simulink model "Ex4_IC"  (R2021a)
settings: Solver=VariableStepAuto  StartTime=0.0  StopTime=10.0  RelTol=1e-3
undefined symbols (not defined in the file): fdesignblkfcn, gcbh
libraries: dsparch4 x1
settings Model: Creator=gferr  LastModifiedBy=gferr

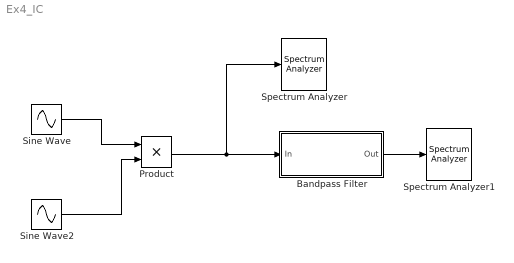
== system Ex4_IC ==
  Bandpass Filter : Subsystem  DialogController=fdesignblkfcn  InitFcn=fdesignblkfcn(gcbh, {'InitFcn'});  mask(Bandpass Filter){}
      mask help: Design a bandpass filter
      settings: CopyFcn=fdesignblkfcn(gcbh, {'CopyFcn'});
      mask Help: helpview(mapfilelocation('dsp'), 'dspbandpassfilter');
      mask Display: disp('Bandpass');
  Product : Product
  Sine Wave : Sin  Frequency=20e9  SampleTime=5e-11
  Sine Wave2 : Sin  Frequency=3.5e9  SampleTime=5e-11
  Spectrum Analyzer : SpectrumAnalyzer
  Spectrum Analyzer1 : SpectrumAnalyzer
  wires:
  Product/1 -> Bandpass Filter/1(In), Spectrum Analyzer/1
  Sine Wave2/1 -> Product/2
  Sine Wave/1 -> Product/1
  Bandpass Filter/1(Out) -> Spectrum Analyzer1/1

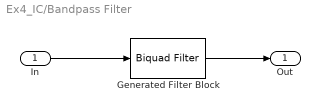
== system Ex4_IC/Bandpass Filter ==
  In : Inport
  Generated Filter Block : dsparch4/Biquad Filter  Tag=BlockMethodSubSystem  FilterSource=Dialog parameters  CoeffSource=Specify via dialog  FilterObject=BQF  IIRFiltStruct=Direct form II  BiQuadCoeffs=[0.00966146652633205656 0 -0.00966146652633205656 1 -0.893732410630936891 0.984405274774847627;0.00330714192391191354 0 -0.00330714192391191354 1 -0.880244202993088365 0.984346529334988007;0.0166040427440116885 0 -0.0166040427440116885 1 -0.907405547432020732 0.996135049550237905;0.0114751093240028565 0 -0.0114751093240028565 1 -0.876964852267980266 0.996102065629321465;0.00541103985322967471 0 -0.00541103985322967471 1 -0.886239861407497886 0.982673189944245795;0.0145645545686283809 0 -0.0145645545686283809 1 -0.90127316214514086 0.989198862457340899;0.560237305861974177 0 -0.560237305861974177 1 -0.876924947595652982 0.989125259648044874]  ScaleValues=[0.0139251488583646554;1;1;1;1;1;1;1]  IC=0  ICnum=0  ICden=0  a0Flag=Warning  optimizeScaleValues=off  ScaleValueMode=Specify via input port (g)  InputProcessing=Columns as channels (frame based)  roundingMode=Floor  overflowMode=off  scaleValueFracLength=14  denProdOutputFracLength=30  denAccumFracLength=30  secondMemoryFracLength=15
  Out : Outport  VectorParamsAs1DForOutWhenUnconnected=off
  wires:
  In/1 -> Generated Filter Block/1
  Generated Filter Block/1 -> Out/1
